simulink model "correct"  (R2024b)
settings: Solver=FixedStepAuto  StartTime=0.0  StopTime=10.0  FixedStep=1  RelTol=1e-3
undefined symbols (not defined in the file): C, Vk
settings Model: Creator=54238  LastModifiedBy=54238

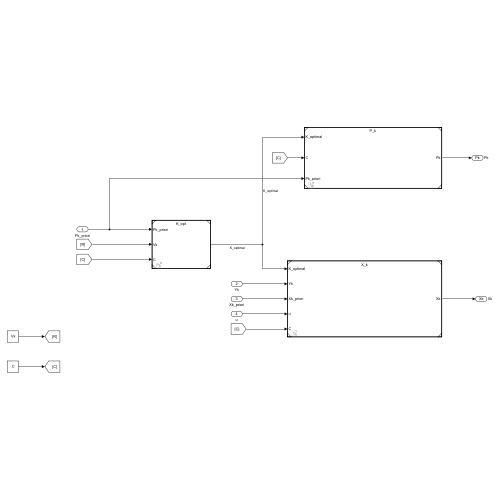
[thumbnail: Simulink's stored preview of the top-level diagram]
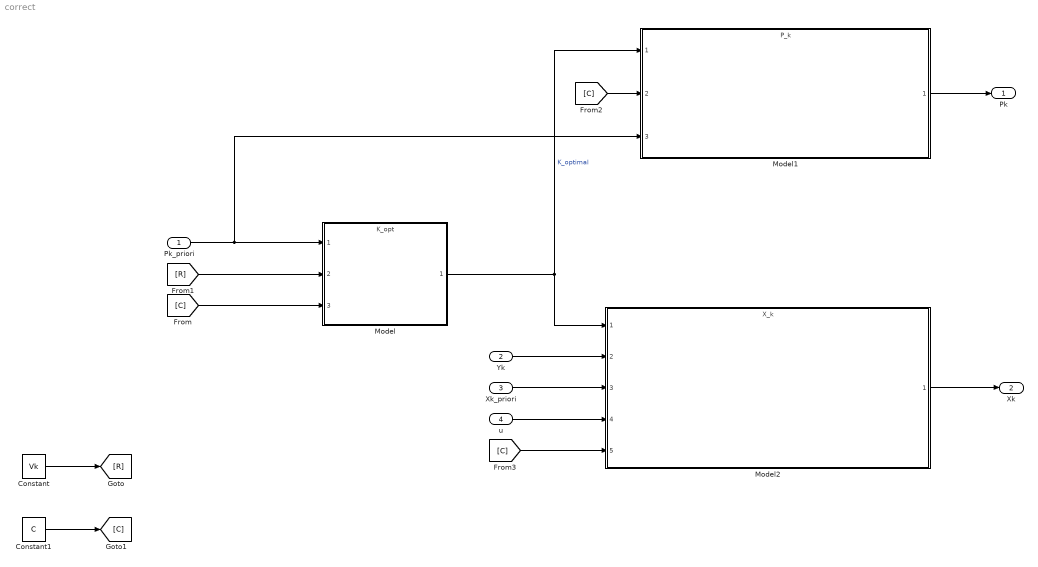
== system correct ==
  Pk_priori : Inport  PortDimensions=[4,4]
  Yk : Inport  Port=2  PortDimensions=[2,1]
  Xk_priori : Inport  Port=3  PortDimensions=[4,1]
  u : Inport  Port=4  PortDimensions=[2,1]
  Constant : Constant  Value=Vk
  Constant1 : Constant  Value=C
  Model : ModelReference  ModelNameDialog=K_opt.slx  SimulationMode=Normal  ModelReferenceVersion=1.3
  Model1 : ModelReference  ModelNameDialog=P_k.slx  SimulationMode=Normal  ModelReferenceVersion=1.5
  Model2 : ModelReference  ModelNameDialog=X_k.slx  SimulationMode=Normal  ModelReferenceVersion=1.2
  Pk : Outport  SignalName=Pk  PortDimensions=[4,4]
  Xk : Outport  Port=2  SignalName=Xk  PortDimensions=[4,1]
  wires:
  [R] -> Model/2
  [C] -> Model/3
  Model/1 -> Model1/1, Model2/1  "K_optimal"
  [C] -> Model1/2
  u/1 -> Model2/4
  Xk_priori/1 -> Model2/3
  [C] -> Model2/5
  Yk/1 -> Model2/2
  Pk_priori/1 -> Model1/3, Model/1
  Constant/1 -> [R]
  Model1/1 -> Pk/1
  Constant1/1 -> [C]
  Model2/1 -> Xk/1
